simulink model "V1_Grid_Forming_corrected_dq_2022"  (R2022b)
settings: Solver=VariableStepAuto  StartTime=0.0  StopTime=2000e-3  RelTol=1e-3
InitFcn:
  | %% Initialize twist parameters
  | source_V = 0;
  | Ts = 1e-7;
  | 
  | % set the PID parameters
  | Kp = 0.000215;
  | Ti = 7.5175e-5;
  | Td = 0.0;
  | N  = 0.0;
  | Kd = 0.0;
  | 
  | 
  | %Low side parameters
  | twist_low_side_L = 33e-6;
  | twist_low_side_rL = 20e-3; %Modified
  | twist_low_side_C = 47e-6 + 3*4.7e-6;
  | twist_low_side_C_electrolytic = 47e-6;
  | twist_low_side_C_ceramic = 3*4.7e-6;
  | twist_low_side_rC = 700e-3;
  | twist_low_side_rC_ceramic = 0;
  | twist_low_side_adc_R = 150e3+470;
  | 
  | %High side parameters
  | twist_high_side_C = 33e-6*4 + 4.7e-6*12;
  | twist_high_side_rC = 0.1;
  | twist_high_side_adc_R = 1/(1/2e6 + 1/2e6 + 1/(330e3+5.6e3));
  | twist_high_side_feeder_R = 47e3+4.7e3;
  | R_parallel = 1/(1/twist_high_side_adc_R + 1/twist_high_side_feeder_R);
  | tau_VCC = 0.204;
  | tau_desactive = 0.2;
  | twist_R_VCC = (tau_VCC/twist_high_side_C  - twist_high_side_rC)/(1-(tau_VCC/twist_high_side_C - twist_high_side_rC)/R_parallel);
  | 
  | %High side feeder current
  | %load('feeder_current.mat');
  | feeder_VHigh_min = 12;
  | feeder_VHigh_spacing = 6;
  | feeder_duty_min = 0.1;
  | feeder_duty_spacing = 0.4;
  | feeder_Vth_stop = 8.9;
  | feeder_Vth_start = 9.7;
  | feeder_current_upper_rate_limit = 0.386/(20e-3);
  | feeder_current_lower_rate_limit = -500;
  | 
  | %MOSFET parameters
  | twist_FET_Ron = 0.016;
  | twist_FET_Lon = 0;
  | twist_FET_Rd = 0.006;
  | twist_FET_Vf = 0.7;
  | twist_FET_Rs = 1e10;
  | twist_FET_Cs = inf;
  | twist_FET_Clow_Ron = 220e-3;
  | twist_FET_Clow_Rd = 45e-3; %Modified
  | twist_FET_Clow_Vf = 0.7; %Modified
  | 
  | 
  | %Schottky diode parameters
  | twist_shottky_Ron = 0.48; %Modified
  | twist_shottky_Vf = 0.28; %Modified
  | twist_shottky_Rs = 1e10;
  | twist_shottky_Cs = inf;
  | 
  | %PWM generation
  | twist_freq_switching = 200e3; %carry switching frequency
  | twist_period_switching = 1/twist_freq_switching; %carry switching period
  | twist_pwm_resolution = 100e-9; %resolution of the PWM generator - increasing it reduces simulation time
  | twist_duty_cycle_min = 0; %minimum duty cycle
  | twist_duty_cycle_max = 1; %maximum duty cycle
  | twist_dead_time = 200e-9; %duty cycle positive dead time
  | 
  | % Initialize times and frequencies
  | twist_freq_data_sampling = 20e3; %data sampling frequency
  | twist_data_sampling_period = 1/twist_freq_data_sampling; %data sampling delay
  | twist_data_acquisition_delay = 50e-9; %data acquisition at the peak of the carry
undefined symbols (not defined in the file): DiscIntNeverNeededParam, gcbh, sps_rtmsupport, twist_low_side_lC
libraries: spsSeriesRLCBranchLib x13, spsTriangleGeneratorLib x6, spsMosfetLib x6, slpidlib x4, spsCurrentMeasurementLib x4, spsControlledCurrentSourceLib x3, spsVoltageMeasurementLib x3, eeTransforms x2, dspstat3 x2, spsIdealSwitchLib x2, spsDiodeLib x2, spspowerguiLib x2
(part 1 of 2)
settings Model: Creator=ABS_Lab  LastModifiedBy=ABS_Lab

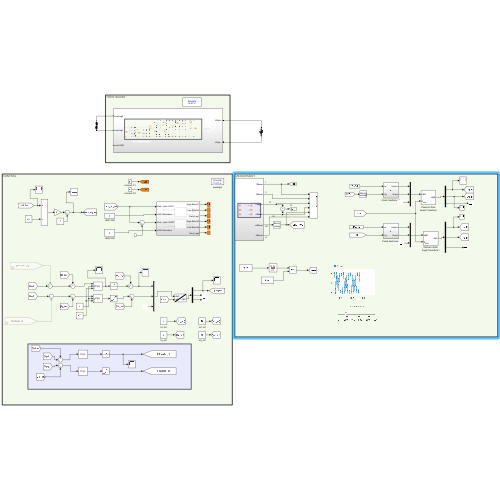
[thumbnail: Simulink's stored preview of the top-level diagram]
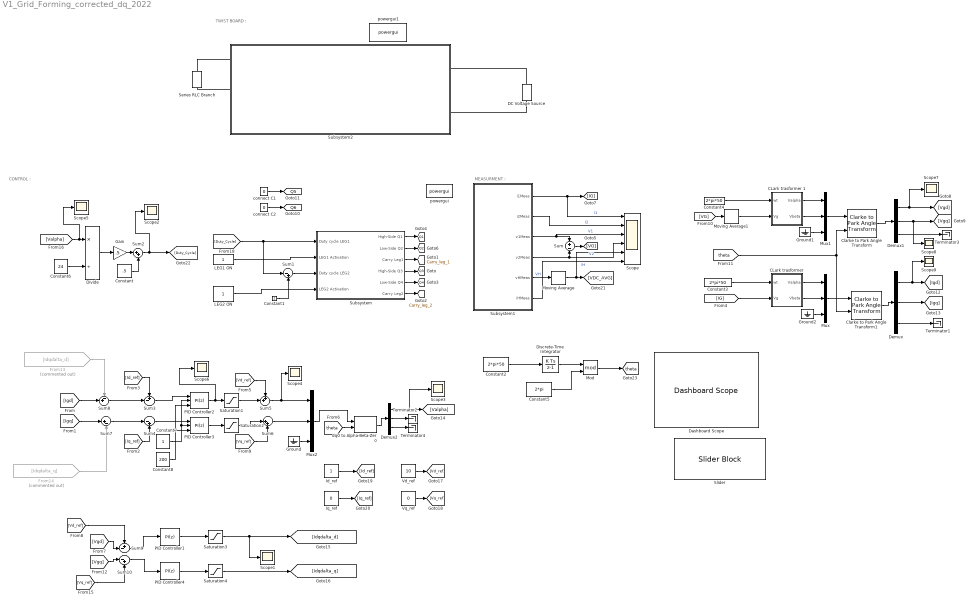
== system V1_Grid_Forming_corrected_dq_2022 ==
  note: TWIST BOARD :
  note: CONTROL :
  note: MEASURMENT :
  "CLark trasformer " : Subsystem
  CLark trasformer 1 : Subsystem
  Clarke to Park Angle Transform : eeTransforms/Clarke to Park Angle Transform  AxisAlignment=Q-axis
      settings: LibrarySourceBlock=|
      | ee_sl_lib/Mathematical
      | Transforms/Clarke to Park
      | Angle Transform
  Clarke to Park Angle Transform1 : eeTransforms/Clarke to Park Angle Transform  AxisAlignment=Q-axis
      settings: LibrarySourceBlock=|
      | ee_sl_lib/Mathematical
      | Transforms/Clarke to Park
      | Angle Transform
  Constant : Constant  Value=.5
  Constant1 : Constant
  Constant2 : Constant  Value=2*pi*50
  Constant3 : Constant  Value=2*pi*50
  Constant4 : Constant  Value=2*pi*50
  Constant5 : Constant  Value=2*pi
  Constant6 : Constant  Value=24
  Constant7 : Constant
  Constant8 : Constant  Value=200
  DC Voltage Source : spsDCVoltageSourceLib/DC Voltage Source  Amplitude=24  Measurements=None
  Dashboard Scope : DashboardScope  TimeSpan=0.080000000000000002  Ymin=-20  Ymax=20
  Demux : Demux  Outputs=3
  Demux1 : Demux  Outputs=3
  Demux2 : Demux  Outputs=3
  Discrete-Time Integrator : DiscreteIntegrator  SampleTime=-1  ICPrevOutput=DiscIntNeverNeededParam  ICPrevScaledInput=DiscIntNeverNeededParam
  Divide : Product  Inputs=*/
  From13 : From  Commented=on  GotoTag=Idqdalta_d
  From14 : From  Commented=on  GotoTag=Idqdalta_q
  Gain : Gain  Gain=.5
  Ground : Ground
  Ground1 : Ground
  Ground2 : Ground
  Id_ref : Constant
  Iq_ref : Constant  Value=0
  LEG1 ON : Constant
  LEG2 ON : Constant
  Mod : Math  Operator=mod
  Moving Average : dspstat3/Moving Average  Method=Sliding window  ForgettingFactorPort=off  SpecifyWindowLength=on  WindowLength=4  OverlapLength=3  AllowArbitraryInputLength=off  ForgettingFactor=0.9  SimulateUsing=Code generation
  Moving Average1 : dspstat3/Moving Average  Method=Sliding window  ForgettingFactorPort=off  SpecifyWindowLength=on  WindowLength=15  OverlapLength=14  AllowArbitraryInputLength=off  ForgettingFactor=0.9  SimulateUsing=Code generation
  Mux : Mux  Inputs=3
  Mux1 : Mux  Inputs=3
  Mux2 : Mux  Inputs=3
  PID Controller1 : slpidlib/PID Controller  Controller=PI  Form=Parallel  TimeDomain=Discrete-time  UseExternalTs=off  SampleTime=-1  IntegratorMethod=Forward Euler  FilterMethod=Forward Euler  ControllerParametersSource=internal  P=.01  I=3000  UseKiTs=off  D=0  N=100  UseFilter=on  TunerSelectOption=Transfer Function Based (PID Tuner App)  InitialConditionSource=internal  InitialConditionForIntegrator=0  InitialConditionForFilter=0  DifferentiatorICPrevScaledInput=0  ExternalReset=none  TrackingMode=off  Kt=1  LimitOutput=off  SatLimitsSource=internal  UpperSaturationLimit=inf  LowerSaturationLimit=-inf  LinearizeAsGain=on  AntiWindupMode=none  Kb=1  LimitIntegrator=off  UpperIntegratorSaturationLimit=inf  LowerIntegratorSaturationLimit=-inf  POutMin=[]  POutMax=[]  IOutMin=[]  IOutMax=[]  DOutMin=[]  DOutMax=[]  NOutMin=[]  NOutMax=[]  SumOutMin=[]  SumOutMax=[]  SaturationOutMin=[]  SaturationOutMax=[]  PParamMin=[]  PParamMax=[]  IParamMin=[]  IParamMax=[]  DParamMin=[]  DParamMax=[]  NParamMin=[]  NParamMax=[]  KbParamMin=[]  KbParamMax=[]  KtParamMin=[]  KtParamMax=[]  KbOutMin=[]  KbOutMax=[]  KtOutMin=[]  KtOutMax=[]  IntegratorOutMin=[]  IntegratorOutMax=[]  FilterOutMin=[]  FilterOutMax=[]  SumI1OutMin=[]  SumI1OutMax=[]  SumI2OutMin=[]  SumI2OutMax=[]  SumI3OutMin=[]  SumI3OutMax=[]  SumI4OutMin=[]  SumI4OutMax=[]  SumDOutMin=[]  SumDOutMax=[]  DifferentiatorOutMin=[]  DifferentiatorOutMax=[]  FilterDiffOutCoefMin=[]  FilterDiffOutCoefMax=[]  ReciprocalOutMin=[]  ReciprocalOutMax=[]  SumDenOutMin=[]  SumDenOutMax=[]  SumNumOutMin=[]  SumNumOutMax=[]  DivideOutMin=[]  DivideOutMax=[]  UdiffTsProdOutMin=[]  UdiffTsProdOutMax=[]  NTsProdOutMin=[]  NTsProdOutMax=[]  UintegralTsProdOutMin=[]  UintegralTsProdOutMax=[]  UngainTsProdOutMin=[]  UngainTsProdOutMax=[]  ClampingZeroOutDataTypeStr=Inherit: Inherit via back propagation  ClampingZeroOutMin=[]  ClampingZeroOutMax=[]  FilterDenConstantOutDataTypeStr=Inherit: Inherit via back propagation  FilterDenConstantOutMin=[]  FilterDenConstantOutMax=[]  PCopyOutDataTypeStr=Inherit: Inherit via back propagation  PCopyOutMin=[]  PCopyOutMax=[]  NCopyOutDataTypeStr=Inherit: Inherit via back propagation  NCopyOutMin=[]  NCopyOutMax=[]  IntegratorContinuousStateAttributes=''  IntegratorStateMustResolveToSignalObject=off  IntegratorRTWStateStorageClass=Auto  FilterContinuousStateAttributes=''  FilterStateMustResolveToSignalObject=off  FilterRTWStateStorageClass=Auto  ParallelPVariant=InternalParameters  IdealPVariant=Disabled  IVariant=InternalParameters  DVariant=Disabled  IntegratorVariant=Discrete  SatVariant=Disabled  AWVariant=Passthrough  PCopyVariant=Disabled  TRVariant=Disabled  FdbkBlocksVariant=Forward  IdealPFdbkVariant=Disabled  SatFdbkVariant=Disabled  DerivativeFilterVariant=Disabled  NVariant=Disabled  NCopyVariant=Disabled_SignalSpec  FilterICVariant=Disabled  IntegratorICVariant=InternalICs  ExternalResetVariant=Disabled  TRSumVariant=Passthrough  SumFdbkVariant=Disabled  SumVariant=Sum_PI  TsampFilterVariant=InternalTs  TsampNgainVariant=Passthrough  TsampIntegralVariant=Passthrough  ExternalSaturationOutDataTypeStr=Inherit: Same as second input
  PID Controller2 : slpidlib/PID Controller  Controller=PI  Form=Parallel  TimeDomain=Discrete-time  UseExternalTs=off  SampleTime=Ts*1000  IntegratorMethod=Forward Euler  FilterMethod=Forward Euler  ControllerParametersSource=external  P=.1  I=2000  UseKiTs=off  D=0  N=100  UseFilter=on  TunerSelectOption=Transfer Function Based (PID Tuner App)  InitialConditionSource=internal  InitialConditionForIntegrator=0  InitialConditionForFilter=0  DifferentiatorICPrevScaledInput=0  ExternalReset=none  TrackingMode=off  Kt=1  LimitOutput=off  SatLimitsSource=internal  UpperSaturationLimit=inf  LowerSaturationLimit=-inf  LinearizeAsGain=on  AntiWindupMode=none  Kb=1  LimitIntegrator=off  UpperIntegratorSaturationLimit=inf  LowerIntegratorSaturationLimit=-inf  POutMin=[]  POutMax=[]  IOutMin=[]  IOutMax=[]  DOutMin=[]  DOutMax=[]  NOutMin=[]  NOutMax=[]  SumOutMin=[]  SumOutMax=[]  SaturationOutMin=[]  SaturationOutMax=[]  PParamMin=[]  PParamMax=[]  IParamMin=[]  IParamMax=[]  DParamMin=[]  DParamMax=[]  NParamMin=[]  NParamMax=[]  KbParamMin=[]  KbParamMax=[]  KtParamMin=[]  KtParamMax=[]  KbOutMin=[]  KbOutMax=[]  KtOutMin=[]  KtOutMax=[]  IntegratorOutMin=[]  IntegratorOutMax=[]  FilterOutMin=[]  FilterOutMax=[]  SumI1OutMin=[]  SumI1OutMax=[]  SumI2OutMin=[]  SumI2OutMax=[]  SumI3OutMin=[]  SumI3OutMax=[]  SumI4OutMin=[]  SumI4OutMax=[]  SumDOutMin=[]  SumDOutMax=[]  DifferentiatorOutMin=[]  DifferentiatorOutMax=[]  FilterDiffOutCoefMin=[]  FilterDiffOutCoefMax=[]  ReciprocalOutMin=[]  ReciprocalOutMax=[]  SumDenOutMin=[]  SumDenOutMax=[]  SumNumOutMin=[]  SumNumOutMax=[]  DivideOutMin=[]  DivideOutMax=[]  UdiffTsProdOutMin=[]  UdiffTsProdOutMax=[]  NTsProdOutMin=[]  NTsProdOutMax=[]  UintegralTsProdOutMin=[]  UintegralTsProdOutMax=[]  UngainTsProdOutMin=[]  UngainTsProdOutMax=[]  ClampingZeroOutDataTypeStr=Inherit: Inherit via back propagation  ClampingZeroOutMin=[]  ClampingZeroOutMax=[]  FilterDenConstantOutDataTypeStr=Inherit: Inherit via back propagation  FilterDenConstantOutMin=[]  FilterDenConstantOutMax=[]  PCopyOutDataTypeStr=Inherit: Inherit via back propagation  PCopyOutMin=[]  PCopyOutMax=[]  NCopyOutDataTypeStr=Inherit: Inherit via back propagation  NCopyOutMin=[]  NCopyOutMax=[]  IntegratorContinuousStateAttributes=''  IntegratorStateMustResolveToSignalObject=off  IntegratorRTWStateStorageClass=Auto  FilterContinuousStateAttributes=''  FilterStateMustResolveToSignalObject=off  FilterRTWStateStorageClass=Auto  ParallelPVariant=ExternalParameters  IdealPVariant=Disabled  IVariant=ExternalParameters  DVariant=Disabled  IntegratorVariant=Discrete  SatVariant=Disabled  AWVariant=Passthrough  PCopyVariant=Disabled  TRVariant=Disabled  FdbkBlocksVariant=Forward  IdealPFdbkVariant=Disabled  SatFdbkVariant=Disabled  DerivativeFilterVariant=Disabled  NVariant=Disabled  NCopyVariant=Disabled_SignalSpec  FilterICVariant=Disabled  IntegratorICVariant=InternalICs  ExternalResetVariant=Disabled  TRSumVariant=Passthrough  SumFdbkVariant=Disabled  SumVariant=Sum_PI  TsampFilterVariant=InternalTs  TsampNgainVariant=Passthrough  TsampIntegralVariant=Passthrough  ExternalSaturationOutDataTypeStr=Inherit: Same as second input
  PID Controller3 : slpidlib/PID Controller  Controller=PI  Form=Parallel  TimeDomain=Discrete-time  UseExternalTs=off  SampleTime=Ts*1000  IntegratorMethod=Forward Euler  FilterMethod=Forward Euler  ControllerParametersSource=external  P=.1  I=100  UseKiTs=off  D=0  N=100  UseFilter=on  TunerSelectOption=Transfer Function Based (PID Tuner App)  InitialConditionSource=internal  InitialConditionForIntegrator=0  InitialConditionForFilter=0  DifferentiatorICPrevScaledInput=0  ExternalReset=none  TrackingMode=off  Kt=1  LimitOutput=off  SatLimitsSource=internal  UpperSaturationLimit=inf  LowerSaturationLimit=-inf  LinearizeAsGain=on  AntiWindupMode=none  Kb=1  LimitIntegrator=off  UpperIntegratorSaturationLimit=inf  LowerIntegratorSaturationLimit=-inf  POutMin=[]  POutMax=[]  IOutMin=[]  IOutMax=[]  DOutMin=[]  DOutMax=[]  NOutMin=[]  NOutMax=[]  SumOutMin=[]  SumOutMax=[]  SaturationOutMin=[]  SaturationOutMax=[]  PParamMin=[]  PParamMax=[]  IParamMin=[]  IParamMax=[]  DParamMin=[]  DParamMax=[]  NParamMin=[]  NParamMax=[]  KbParamMin=[]  KbParamMax=[]  KtParamMin=[]  KtParamMax=[]  KbOutMin=[]  KbOutMax=[]  KtOutMin=[]  KtOutMax=[]  IntegratorOutMin=[]  IntegratorOutMax=[]  FilterOutMin=[]  FilterOutMax=[]  SumI1OutMin=[]  SumI1OutMax=[]  SumI2OutMin=[]  SumI2OutMax=[]  SumI3OutMin=[]  SumI3OutMax=[]  SumI4OutMin=[]  SumI4OutMax=[]  SumDOutMin=[]  SumDOutMax=[]  DifferentiatorOutMin=[]  DifferentiatorOutMax=[]  FilterDiffOutCoefMin=[]  FilterDiffOutCoefMax=[]  ReciprocalOutMin=[]  ReciprocalOutMax=[]  SumDenOutMin=[]  SumDenOutMax=[]  SumNumOutMin=[]  SumNumOutMax=[]  DivideOutMin=[]  DivideOutMax=[]  UdiffTsProdOutMin=[]  UdiffTsProdOutMax=[]  NTsProdOutMin=[]  NTsProdOutMax=[]  UintegralTsProdOutMin=[]  UintegralTsProdOutMax=[]  UngainTsProdOutMin=[]  UngainTsProdOutMax=[]  ClampingZeroOutDataTypeStr=Inherit: Inherit via back propagation  ClampingZeroOutMin=[]  ClampingZeroOutMax=[]  FilterDenConstantOutDataTypeStr=Inherit: Inherit via back propagation  FilterDenConstantOutMin=[]  FilterDenConstantOutMax=[]  PCopyOutDataTypeStr=Inherit: Inherit via back propagation  PCopyOutMin=[]  PCopyOutMax=[]  NCopyOutDataTypeStr=Inherit: Inherit via back propagation  NCopyOutMin=[]  NCopyOutMax=[]  IntegratorContinuousStateAttributes=''  IntegratorStateMustResolveToSignalObject=off  IntegratorRTWStateStorageClass=Auto  FilterContinuousStateAttributes=''  FilterStateMustResolveToSignalObject=off  FilterRTWStateStorageClass=Auto  ParallelPVariant=ExternalParameters  IdealPVariant=Disabled  IVariant=ExternalParameters  DVariant=Disabled  IntegratorVariant=Discrete  SatVariant=Disabled  AWVariant=Passthrough  PCopyVariant=Disabled  TRVariant=Disabled  FdbkBlocksVariant=Forward  IdealPFdbkVariant=Disabled  SatFdbkVariant=Disabled  DerivativeFilterVariant=Disabled  NVariant=Disabled  NCopyVariant=Disabled_SignalSpec  FilterICVariant=Disabled  IntegratorICVariant=InternalICs  ExternalResetVariant=Disabled  TRSumVariant=Passthrough  SumFdbkVariant=Disabled  SumVariant=Sum_PI  TsampFilterVariant=InternalTs  TsampNgainVariant=Passthrough  TsampIntegralVariant=Passthrough  ExternalSaturationOutDataTypeStr=Inherit: Same as second input
  PID Controller4 : slpidlib/PID Controller  Controller=PI  Form=Parallel  TimeDomain=Discrete-time  UseExternalTs=off  SampleTime=-1  IntegratorMethod=Forward Euler  FilterMethod=Forward Euler  ControllerParametersSource=internal  P=.01  I=3000  UseKiTs=off  D=0  N=100  UseFilter=on  TunerSelectOption=Transfer Function Based (PID Tuner App)  InitialConditionSource=internal  InitialConditionForIntegrator=0  InitialConditionForFilter=0  DifferentiatorICPrevScaledInput=0  ExternalReset=none  TrackingMode=off  Kt=1  LimitOutput=off  SatLimitsSource=internal  UpperSaturationLimit=inf  LowerSaturationLimit=-inf  LinearizeAsGain=on  AntiWindupMode=none  Kb=1  LimitIntegrator=off  UpperIntegratorSaturationLimit=inf  LowerIntegratorSaturationLimit=-inf  POutMin=[]  POutMax=[]  IOutMin=[]  IOutMax=[]  DOutMin=[]  DOutMax=[]  NOutMin=[]  NOutMax=[]  SumOutMin=[]  SumOutMax=[]  SaturationOutMin=[]  SaturationOutMax=[]  PParamMin=[]  PParamMax=[]  IParamMin=[]  IParamMax=[]  DParamMin=[]  DParamMax=[]  NParamMin=[]  NParamMax=[]  KbParamMin=[]  KbParamMax=[]  KtParamMin=[]  KtParamMax=[]  KbOutMin=[]  KbOutMax=[]  KtOutMin=[]  KtOutMax=[]  IntegratorOutMin=[]  IntegratorOutMax=[]  FilterOutMin=[]  FilterOutMax=[]  SumI1OutMin=[]  SumI1OutMax=[]  SumI2OutMin=[]  SumI2OutMax=[]  SumI3OutMin=[]  SumI3OutMax=[]  SumI4OutMin=[]  SumI4OutMax=[]  SumDOutMin=[]  SumDOutMax=[]  DifferentiatorOutMin=[]  DifferentiatorOutMax=[]  FilterDiffOutCoefMin=[]  FilterDiffOutCoefMax=[]  ReciprocalOutMin=[]  ReciprocalOutMax=[]  SumDenOutMin=[]  SumDenOutMax=[]  SumNumOutMin=[]  SumNumOutMax=[]  DivideOutMin=[]  DivideOutMax=[]  UdiffTsProdOutMin=[]  UdiffTsProdOutMax=[]  NTsProdOutMin=[]  NTsProdOutMax=[]  UintegralTsProdOutMin=[]  UintegralTsProdOutMax=[]  UngainTsProdOutMin=[]  UngainTsProdOutMax=[]  ClampingZeroOutDataTypeStr=Inherit: Inherit via back propagation  ClampingZeroOutMin=[]  ClampingZeroOutMax=[]  FilterDenConstantOutDataTypeStr=Inherit: Inherit via back propagation  FilterDenConstantOutMin=[]  FilterDenConstantOutMax=[]  PCopyOutDataTypeStr=Inherit: Inherit via back propagation  PCopyOutMin=[]  PCopyOutMax=[]  NCopyOutDataTypeStr=Inherit: Inherit via back propagation  NCopyOutMin=[]  NCopyOutMax=[]  IntegratorContinuousStateAttributes=''  IntegratorStateMustResolveToSignalObject=off  IntegratorRTWStateStorageClass=Auto  FilterContinuousStateAttributes=''  FilterStateMustResolveToSignalObject=off  FilterRTWStateStorageClass=Auto  ParallelPVariant=InternalParameters  IdealPVariant=Disabled  IVariant=InternalParameters  DVariant=Disabled  IntegratorVariant=Discrete  SatVariant=Disabled  AWVariant=Passthrough  PCopyVariant=Disabled  TRVariant=Disabled  FdbkBlocksVariant=Forward  IdealPFdbkVariant=Disabled  SatFdbkVariant=Disabled  DerivativeFilterVariant=Disabled  NVariant=Disabled  NCopyVariant=Disabled_SignalSpec  FilterICVariant=Disabled  IntegratorICVariant=InternalICs  ExternalResetVariant=Disabled  TRSumVariant=Passthrough  SumFdbkVariant=Disabled  SumVariant=Sum_PI  TsampFilterVariant=InternalTs  TsampNgainVariant=Passthrough  TsampIntegralVariant=Passthrough  ExternalSaturationOutDataTypeStr=Inherit: Same as second input
  Saturation1 : Saturate  UpperLimit=24  LowerLimit=-24
  Saturation2 : Saturate  UpperLimit=24  LowerLimit=-24
  Saturation3 : Saturate  UpperLimit=10  LowerLimit=-10
  Saturation4 : Saturate  UpperLimit=10  LowerLimit=-10
  Scope : Scope  NumInputPorts=6
  Scope{1..9} (9 alike) : Scope
  Series RLC Branch : spsSeriesRLCBranchLib/Series RLC Branch  LConnTagsString=__new0  RConnTagsString=__new0  BranchType=RL  Resistance=10  Inductance=100e-8  SetiL0=off  InitialCurrent=0  Capacitance=1e-6  Setx0=off  InitialVoltage=0  Measurements=None
  Slider : SliderBlock  ScaleMax=1000
  Subsystem : Subsystem
  Subsystem1 : Subsystem
  Subsystem2 : Subsystem
  Sum : Sum  Inputs=+|-
  Sum1 : Sum  Inputs=|-+
  Sum10 : Sum  Inputs=|-+
  Sum2 : Sum  Inputs=|++
  Sum3 : Sum  Inputs=+-|
  Sum4 : Sum  Inputs=|-+
  Sum5 : Sum  Inputs=++|
  Sum6 : Sum  Inputs=|++
  Sum7 : Sum  Inputs=|+-
  Sum8 : Sum  Inputs=-+|
  Sum9 : Sum  Inputs=+-|
  Terminator{1..4} (4 alike) : Terminator
  Vd_ref : Constant  Value=10
  Vq_ref : Constant  Value=0
  connect C1 : Constant  Value=0
  connect C2 : Constant  Value=0
  dq0 to Alpha-Beta-Zero : spsdq0toAlphaBetaZeroLib/dq0 to Alpha-Beta-Zero  Alignment=90 degrees behind phase A axis
  powergui : spspowerguiLib/powergui  Priority=1  SimulationMode=Discrete  SampleTime=Ts  frequency=60  Iterations=50  frequencyindice=0  Pbase=100e6  ErrMax=1e-4  UnitsV=kV  UnitsW=MW  buscounter=0  FunctionMessages=off  echomessages=off  EnableUseOfTLC=off  CurrentSourceSwitches=off  DisableSnubberDevices=off  DisableRonSwitches=off  DisableVfSwitches=off  DisplayEquations=off  AutomaticDiscreteSolvers=off  SolverType=Tustin/Backward Euler (TBE)  Interpol=off  ExternalGateDelay=off  methode=off  Ts=100  x0status=blocks  SPID=on  SwTol=0  HookPort=off  NonlinearTolerance=1e-4  nMaxIteration=100  ContinueOnMaxIteration=off  RestoreLinks=warning  ResistiveCurrentMeasurement=off  Frange=[0:2:500]  Ylog=off  Xlog=on  ShowGrid=off  save=off  variable=ZData  structure=0  ZoomFFT=off  StartTime=0.0  cycles=1  DisplayStyle=1  fundamental=60  FreqAxis=off  MaxFrequency=1000  frequencyindicesteady=1  RmsSteady=1  display=off
  powergui1 : spspowerguiLib/powergui  Priority=1  SimulationMode=Discrete  SampleTime=Ts  frequency=60  Iterations=50  frequencyindice=60  Pbase=100e6  ErrMax=1e-4  UnitsV=kV  UnitsW=MW  buscounter=0  FunctionMessages=off  echomessages=off  EnableUseOfTLC=off  CurrentSourceSwitches=off  DisableSnubberDevices=off  DisableRonSwitches=off  DisableVfSwitches=off  DisplayEquations=off  AutomaticDiscreteSolvers=off  SolverType=Tustin/Backward Euler (TBE)  Interpol=off  ExternalGateDelay=off  methode=off  Ts=100  x0status=blocks  SPID=on  SwTol=0  HookPort=off  NonlinearTolerance=1e-4  nMaxIteration=100  ContinueOnMaxIteration=off  RestoreLinks=warning  ResistiveCurrentMeasurement=off  Frange=[0:2:500]  Ylog=off  Xlog=on  ShowGrid=off  save=off  variable=ZData  structure=0  ZoomFFT=off  StartTime=0.0  cycles=1  DisplayStyle=1  fundamental=60  FreqAxis=off  MaxFrequency=1000  frequencyindicesteady=1  RmsSteady=1  display=off
  tag scope: Carry_leg_1=global, Carry_leg_2=global, Q1=global, Q2=global, Q3=global, Q4=global, Q5=global, Q6=global, theta=global
  wires:
  Sum1/1 -> Subsystem/3(Duty cycle LEG2)
  connect C1/1 -> [Q5]
  LEG1 ON/1 -> Subsystem/2(LEG1 Activation)
  Subsystem/3(Carry Leg1) -> [Carry_leg_1]
  Subsystem1/3(v1Meas) -> Scope/3, Sum/1  "V1"
  LEG2 ON/1 -> Subsystem/4("LEG2 Activation ")
  [Duty_Cycle] -> Sum1/1, Subsystem/1(Duty cycle LEG1)
  connect C2/1 -> [Q6]
  Subsystem/2(Low-Side Q2) -> [Q2]
  Subsystem/5(Low-Side Q4) -> [Q4]
  Subsystem1/6(iHMeas) -> Scope/6  "IH"
  Subsystem/1(High-Side Q1) -> [Q1]
  Subsystem/6(Carry Leg2) -> [Carry_leg_2]
  Constant1/1 -> Sum1/2
  Subsystem1/2(i2Meas) -> Scope/2  "I2"
  Subsystem/4(High-Side Q3) -> [Q3]
  Subsystem1/4(v2Meas) -> Scope/4, Sum/2  "V2"
  Demux1/1 -> Scope7/1, [Vgd]
  CLark trasformer 1/2(Vbeta) -> Mux1/2
  [VG] -> Moving Average1/1
  CLark trasformer 1/1(Valpha) -> Mux1/1
  Constant4/1 -> CLark trasformer 1/1(wt)
  Clarke to Park Angle Transform/1 -> Demux1/1
  Mux1/1 -> Clarke to Park Angle Transform/1
  Demux1/2 -> Scope8/1, [Vgq]
  [theta] -> Clarke to Park Angle Transform1/2, Clarke to Park Angle Transform/2
  Demux1/3 -> Terminator3/1
  Sum/1 -> [VG]
  Demux/2 -> [Igq]
  "CLark trasformer "/1(Valpha) -> Mux/1
  Demux/1 -> Scope9/1, [Igd]
  "CLark trasformer "/2(Vbeta) -> Mux/2
  Constant3/1 -> "CLark trasformer "/1(wt)
  Demux/3 -> Terminator1/1
  Clarke to Park Angle Transform1/1 -> Demux/1
  [IG] -> "CLark trasformer "/2(Vg)
  Mux/1 -> Clarke to Park Angle Transform1/1
  Subsystem1/1(i1Meas) -> Scope/1, [IG]  "I1"
  Sum7/1 -> Sum4/1
  Sum5/1 -> Scope4/1, Mux2/1
  Saturation2/1 -> Sum6/1
  From14/1 -> Sum7/2
  Demux2/2 -> Terminator2/1
  Sum6/1 -> Mux2/2
  Saturation1/1 -> Sum5/2
  PID Controller3/1 -> Saturation2/1
  Demux2/1 -> Scope3/1, [Valpha]
  Sum4/1 -> PID Controller3/1
  Mux2/1 -> dq0 to Alpha-Beta-Zero/1
  Sum3/1 -> PID Controller2/1
  dq0 to Alpha-Beta-Zero/1 -> Demux2/1
  From13/1 -> Sum8/1
  Sum8/1 -> Sum3/2
  [theta] -> dq0 to Alpha-Beta-Zero/2
  Demux2/3 -> Terminator4/1
  PID Controller2/1 -> Scope6/1, Saturation1/1
  [Igd] -> Sum8/2
  [Igq] -> Sum7/1
  [Vd_ref] -> Sum9/1
  PID Controller1/1 -> Saturation3/1
  Saturation3/1 -> Scope1/1, [Idqdalta_d]
  PID Controller4/1 -> Saturation4/1
  Saturation4/1 -> [Idqdalta_q]
  Sum9/1 -> PID Controller1/1
  [Vgd] -> Sum9/2
  [Vgq] -> Sum10/1
  Sum10/1 -> PID Controller4/1
  [Vq_ref] -> Sum10/2
  Vd_ref/1 -> [Vd_ref]
  Vq_ref/1 -> [Vq_ref]
  Id_ref/1 -> [Id_ref]
  Iq_ref/1 -> [Iq_ref]
  [Id_ref] -> Sum3/1
  [Iq_ref] -> Sum4/2
  [Vd_ref] -> Sum5/1
  Ground/1 -> Mux2/3
  [Vq_ref] -> Sum6/2
  [Valpha] -> Scope5/1, Divide/1
  Subsystem1/5(vHMeas) -> Moving Average/1  "VH"
  Moving Average/1 -> Scope/5, [VDC_AVG]
  Constant6/1 -> Divide/2
  Divide/1 -> Gain/1
  Gain/1 -> Sum2/1
  Constant/1 -> Sum2/2
  Sum2/1 -> Scope2/1, [Duty_Cycle]
  Ground1/1 -> Mux1/3
  Ground2/1 -> Mux/3
  Mod/1 -> [theta]
  Discrete-Time Integrator/1 -> Mod/1
  Constant2/1 -> Discrete-Time Integrator/1
  Constant5/1 -> Mod/2
  Moving Average1/1 -> CLark trasformer 1/2(Vg)
  Constant7/1 -> PID Controller3/2, PID Controller2/2
  Constant8/1 -> PID Controller3/3, PID Controller2/3
  connections:
  DC Voltage Source/RConn1 -- Subsystem2/RConn1
  Series RLC Branch/LConn1 -- Subsystem2/LConn1
  Subsystem2/LConn2 -- Series RLC Branch/RConn1
  DC Voltage Source/LConn1 -- Subsystem2/RConn2

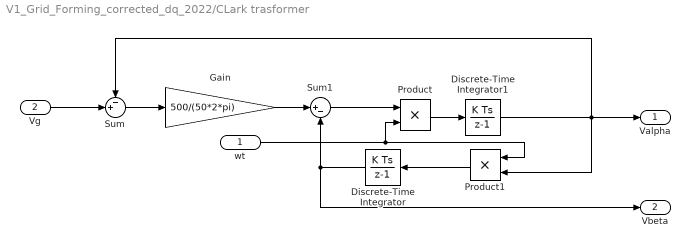
== system V1_Grid_Forming_corrected_dq_2022/CLark trasformer  ==
  wt : Inport
  Vg : Inport  Port=2
  Discrete-Time Integrator : DiscreteIntegrator  SampleTime=Ts*1000  ICPrevOutput=DiscIntNeverNeededParam  ICPrevScaledInput=DiscIntNeverNeededParam
  Discrete-Time Integrator1 : DiscreteIntegrator  SampleTime=Ts*1000  ICPrevOutput=DiscIntNeverNeededParam  ICPrevScaledInput=DiscIntNeverNeededParam
  Gain : Gain  Gain=500/(50*2*pi)
  Product : Product
  Product1 : Product
  Sum : Sum  Inputs=-+|
  Sum1 : Sum  Inputs=|+-
  Valpha : Outport
  Vbeta : Outport  Port=2
  wires:
  Product/1 -> Discrete-Time Integrator1/1
  Discrete-Time Integrator1/1 -> Valpha/1, Product1/2, Sum/1
  Discrete-Time Integrator/1 -> Vbeta/1, Sum1/2
  Gain/1 -> Sum1/1
  wt/1 -> Product1/1, Product/2
  Sum/1 -> Gain/1
  Sum1/1 -> Product/1
  Product1/1 -> Discrete-Time Integrator/1
  Vg/1 -> Sum/2

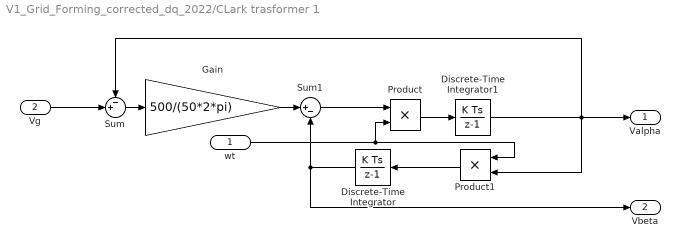
== system V1_Grid_Forming_corrected_dq_2022/CLark trasformer 1 ==
  wt : Inport
  Vg : Inport  Port=2
  Discrete-Time Integrator : DiscreteIntegrator  SampleTime=Ts*1e3  ICPrevOutput=DiscIntNeverNeededParam  ICPrevScaledInput=DiscIntNeverNeededParam
  Discrete-Time Integrator1 : DiscreteIntegrator  SampleTime=Ts*1e3  ICPrevOutput=DiscIntNeverNeededParam  ICPrevScaledInput=DiscIntNeverNeededParam
  Gain : Gain  Gain=500/(50*2*pi)
  Product : Product
  Product1 : Product
  Sum : Sum  Inputs=-+|
  Sum1 : Sum  Inputs=|+-
  Valpha : Outport
  Vbeta : Outport  Port=2
  wires:
  Vg/1 -> Sum/2
  Product1/1 -> Discrete-Time Integrator/1
  Sum1/1 -> Product/1
  Sum/1 -> Gain/1
  wt/1 -> Product/2, Product1/1
  Gain/1 -> Sum1/1
  Discrete-Time Integrator/1 -> Sum1/2, Vbeta/1
  Discrete-Time Integrator1/1 -> Sum/1, Product1/2, Valpha/1
  Product/1 -> Discrete-Time Integrator1/1

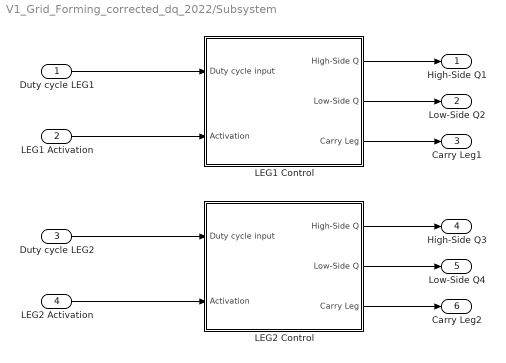
== system V1_Grid_Forming_corrected_dq_2022/Subsystem ==
  Duty cycle LEG1 : Inport
  LEG1 Activation : Inport  Port=2
  Duty cycle LEG2 : Inport  Port=3
  "LEG2 Activation " : Inport  Port=4
  "LEG1 Control " : Subsystem
  LEG2 Control : Subsystem
  High-Side Q1 : Outport
  Low-Side Q2 : Outport  Port=2
  Carry Leg1 : Outport  Port=3
  High-Side Q3 : Outport  Port=4
  Low-Side Q4 : Outport  Port=5
  Carry Leg2 : Outport  Port=6
  wires:
  "LEG1 Control "/3(Carry Leg) -> Carry Leg1/1
  LEG2 Control/1(High-Side Q) -> High-Side Q3/1
  Duty cycle LEG1/1 -> "LEG1 Control "/1(Duty cycle input)
  Duty cycle LEG2/1 -> LEG2 Control/1(Duty cycle input)
  LEG1 Activation/1 -> "LEG1 Control "/2(Activation)
  LEG2 Control/2(Low-Side Q) -> Low-Side Q4/1
  "LEG2 Activation "/1 -> LEG2 Control/2(Activation)
  LEG2 Control/3(Carry Leg) -> Carry Leg2/1
  "LEG1 Control "/1(High-Side Q) -> High-Side Q1/1
  "LEG1 Control "/2(Low-Side Q) -> Low-Side Q2/1

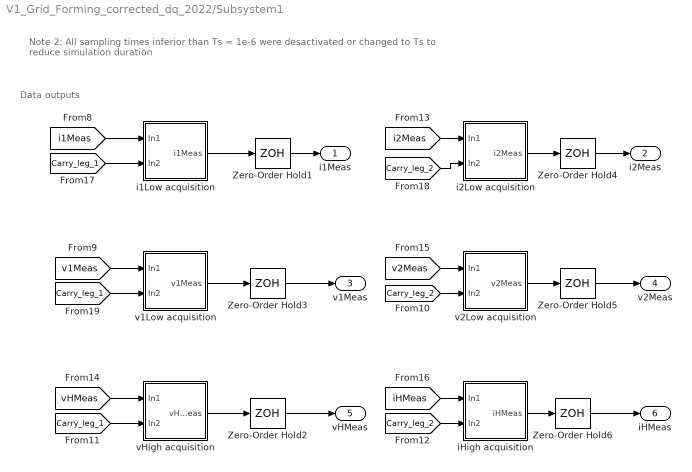
== system V1_Grid_Forming_corrected_dq_2022/Subsystem1 ==
  note: Note 2:
      | All sampling times inferior than Ts = 1e-6 were desactivated or changed to Ts to reduce simulation duration
  note: Data outputs
  Zero-Order Hold{1..6} (6 alike) : ZeroOrderHold  SampleTime=twist_data_sampling_period
  i1Low acquisition : Subsystem
  i2Low acquisition : Subsystem
  iHigh acquisition : Subsystem
  v1Low acquisition : Subsystem
  v2Low acquisition : Subsystem
  vHigh acquisition : Subsystem
  i1Meas : Outport
  i2Meas : Outport  Port=2
  v1Meas : Outport  Port=3
  v2Meas : Outport  Port=4
  vHMeas : Outport  Port=5
  iHMeas : Outport  Port=6
  wires:
  [v2Meas] -> v2Low acquisition/1(In1)
  Zero-Order Hold4/1 -> i2Meas/1
  vHigh acquisition/1(vHMeas) -> Zero-Order Hold2/1
  [i1Meas] -> i1Low acquisition/1(In1)
  [Carry_leg_1] -> vHigh acquisition/2(In2)
  [Carry_leg_1] -> v1Low acquisition/2(In2)
  [vHMeas] -> vHigh acquisition/1(In1)
  [Carry_leg_1] -> i1Low acquisition/2(In2)
  [Carry_leg_2] -> v2Low acquisition/2(In2)
  [v1Meas] -> v1Low acquisition/1(In1)
  Zero-Order Hold5/1 -> v2Meas/1
  [iHMeas] -> iHigh acquisition/1(In1)
  [i2Meas] -> i2Low acquisition/1(In1)
  Zero-Order Hold1/1 -> i1Meas/1
  i2Low acquisition/1(i2Meas) -> Zero-Order Hold4/1
  Zero-Order Hold6/1 -> iHMeas/1
  i1Low acquisition/1(i1Meas) -> Zero-Order Hold1/1
  Zero-Order Hold2/1 -> vHMeas/1
  v1Low acquisition/1(v1Meas) -> Zero-Order Hold3/1
  [Carry_leg_2] -> iHigh acquisition/2(In2)
  [Carry_leg_2] -> i2Low acquisition/2(In2)
  Zero-Order Hold3/1 -> v1Meas/1
  iHigh acquisition/1(iHMeas) -> Zero-Order Hold6/1
  v2Low acquisition/1(v2Meas) -> Zero-Order Hold5/1

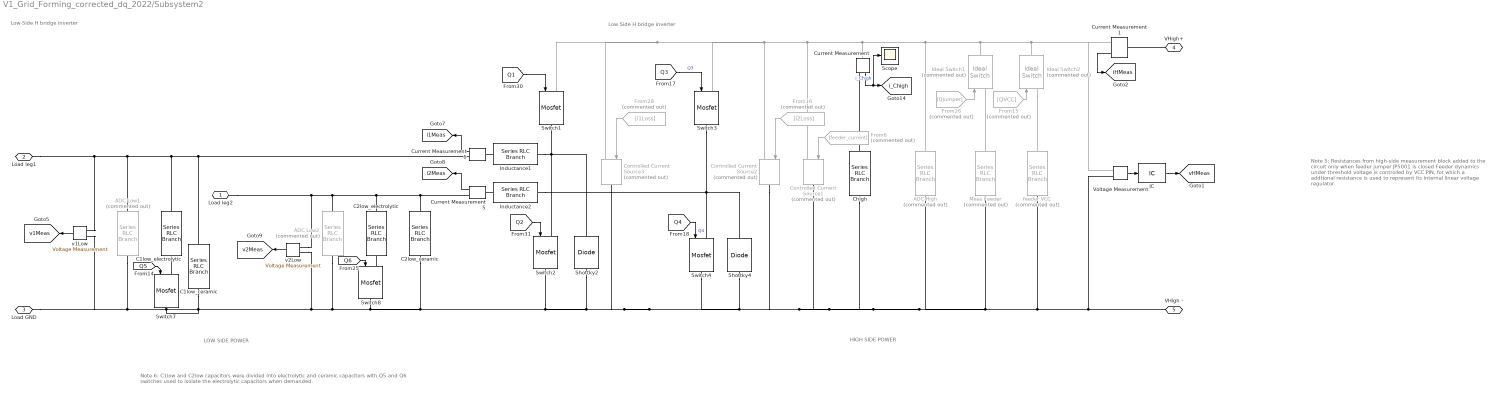
== system V1_Grid_Forming_corrected_dq_2022/Subsystem2 ==
  note: Note 5:
      |
      | Resistances from high-side measurement block added to the circuit only when feeder jumper JP5001 is closed
      |
      | Feeder dynamics under threshold voltage is controlled by VCC PIN, for which a addtional resistance is used to represent its internal linear voltage regulator
  note: Note 6:
      | C1low and C2low capacitors were divided into electrolytic and ceramic capacitors with Q5 and Q6 switches used to isolate the electrolytic capacitors when demanded.
  note: Low Side H bridge inverter
  note: LOW SIDE POWER
  note: HIGH SIDE POWER
  note: Low-Side H bridge inverter
  ADC High : spsSeriesRLCBranchLib/Series RLC Branch  Commented=on  LConnTagsString=__new0  RConnTagsString=__new0  BranchType=R  Resistance=twist_high_side_adc_R  Inductance=twist_low_side_L  SetiL0=off  InitialCurrent=0  Capacitance=1e-6  Setx0=off  InitialVoltage=0  Measurements=None
  ADC Low1 : spsSeriesRLCBranchLib/Series RLC Branch  Commented=on  LConnTagsString=__new0  RConnTagsString=__new0  BranchType=R  Resistance=twist_low_side_adc_R  Inductance=twist_low_side_L  SetiL0=off  InitialCurrent=0  Capacitance=1e-6  Setx0=off  InitialVoltage=0  Measurements=Branch voltage
  ADC Low2 : spsSeriesRLCBranchLib/Series RLC Branch  Commented=on  LConnTagsString=__new0  RConnTagsString=__new0  BranchType=R  Resistance=twist_low_side_adc_R  Inductance=twist_low_side_L  SetiL0=off  InitialCurrent=0  Capacitance=1e-6  Setx0=off  InitialVoltage=0  Measurements=Branch voltage
  C1low_ceramic : spsSeriesRLCBranchLib/Series RLC Branch  LConnTagsString=__new0  RConnTagsString=__new0  BranchType=C  Resistance=twist_low_side_rC  Inductance=1e-3  SetiL0=off  InitialCurrent=0  Capacitance=twist_low_side_C_ceramic  Setx0=off  InitialVoltage=source_V  Measurements=None
  C1low_electrolytic : spsSeriesRLCBranchLib/Series RLC Branch  LConnTagsString=__new0  RConnTagsString=__new0  BranchType=RC  Resistance=twist_low_side_rC  Inductance=twist_low_side_lC  SetiL0=off  InitialCurrent=0  Capacitance=twist_low_side_C_electrolytic  Setx0=off  InitialVoltage=source_V  Measurements=None
  C2low_ceramic : spsSeriesRLCBranchLib/Series RLC Branch  LConnTagsString=__new0  RConnTagsString=__new0  BranchType=C  Resistance=twist_low_side_rC  Inductance=1e-3  SetiL0=off  InitialCurrent=0  Capacitance=twist_low_side_C_ceramic  Setx0=off  InitialVoltage=source_V  Measurements=None
  C2low_electrolytic : spsSeriesRLCBranchLib/Series RLC Branch  LConnTagsString=__new0  RConnTagsString=__new0  BranchType=RC  Resistance=twist_low_side_rC  Inductance=twist_low_side_lC  SetiL0=off  InitialCurrent=0  Capacitance=twist_low_side_C_electrolytic  Setx0=off  InitialVoltage=source_V  Measurements=None
  Chigh : spsSeriesRLCBranchLib/Series RLC Branch  LConnTagsString=__new0  RConnTagsString=__new0  BranchType=RC  Resistance=twist_high_side_rC  Inductance=1e-3  SetiL0=off  InitialCurrent=0  Capacitance=twist_high_side_C  Setx0=on  InitialVoltage=source_V  Measurements=None
  Controlled Current Source1 : spsControlledCurrentSourceLib/Controlled Current Source  Commented=on  Initialize=on  Source_Type=AC  Amplitude=0  Phase=0  Frequency=0  Measurements=None
  Controlled Current Source2 : spsControlledCurrentSourceLib/Controlled Current Source  Commented=on  Initialize=on  Source_Type=AC  Amplitude=0  Phase=0  Frequency=0  Measurements=None
  Controlled Current Source3 : spsControlledCurrentSourceLib/Controlled Current Source  Commented=on  Initialize=on  Source_Type=AC  Amplitude=0  Phase=0  Frequency=0  Measurements=None
  Current Measurement{,1,5..6} (4 alike) : spsCurrentMeasurementLib/Current Measurement  PhasorSimulation=off  OutputType=Complex  PSBequivalent=0
  From15 : From  Commented=on  GotoTag=QVCC
  From16 : From  Commented=on  GotoTag=i2Loss
  From26 : From  Commented=on  GotoTag=Qjumper
  From28 : From  Commented=on  GotoTag=i1Loss
  From6 : From  Commented=on  GotoTag=feeder_current
  IC : InitialCondition  Value=source_V
  Ideal Switch1 : spsIdealSwitchLib/Ideal Switch  Commented=on  Ron=0.001  Lon=0  IC=0  Rs=1e5  Cs=inf  Measurements=off
  Ideal Switch2 : spsIdealSwitchLib/Ideal Switch  Commented=on  Ron=0.001  Lon=0  IC=0  Rs=1e5  Cs=inf  Measurements=off
  Inductance1 : spsSeriesRLCBranchLib/Series RLC Branch  LConnTagsString=__new0  RConnTagsString=__new0  BranchType=RL  Resistance=twist_low_side_rL  Inductance=twist_low_side_L  SetiL0=off  InitialCurrent=0  Capacitance=1e-6  Setx0=off  InitialVoltage=0  Measurements=None
  Inductance2 : spsSeriesRLCBranchLib/Series RLC Branch  LConnTagsString=__new0  RConnTagsString=__new0  BranchType=RL  Resistance=twist_low_side_rL  Inductance=twist_low_side_L  SetiL0=off  InitialCurrent=0  Capacitance=1e-6  Setx0=off  InitialVoltage=0  Measurements=None
  Meas Feeder : spsSeriesRLCBranchLib/Series RLC Branch  Commented=on  LConnTagsString=__new0  RConnTagsString=__new0  BranchType=R  Resistance=twist_high_side_feeder_R  Inductance=twist_low_side_L  SetiL0=off  InitialCurrent=0  Capacitance=1e-6  Setx0=off  InitialVoltage=0  Measurements=None
  Scope : Scope
  Shottky2 : spsDiodeLib/Diode  Ron=twist_shottky_Ron  Lon=0  Vf=twist_shottky_Vf  IC=0  UseSnubber=0  Rs=twist_shottky_Rs  Cs=twist_shottky_Cs  Measurements=off
  Shottky4 : spsDiodeLib/Diode  Ron=twist_shottky_Ron  Lon=0  Vf=twist_shottky_Vf  IC=0  UseSnubber=0  Rs=twist_shottky_Rs  Cs=twist_shottky_Cs  Measurements=off
  Switch{1..4} (4 alike) : spsMosfetLib/Mosfet  Ron=twist_FET_Ron  Lon=0  Rd=twist_FET_Rd  Vfd=twist_FET_Vf  IC=0  Rs=twist_FET_Rs  Cs=twist_FET_Cs  Measurements=off
  Switch7 : spsMosfetLib/Mosfet  Ron=twist_FET_Clow_Ron  Lon=0  Rd=twist_FET_Clow_Ron  Vfd=0  IC=0  Rs=twist_FET_Rs  Cs=twist_FET_Cs  Measurements=off
  Switch8 : spsMosfetLib/Mosfet  Ron=twist_FET_Clow_Ron  Lon=0  Rd=twist_FET_Clow_Ron  Vfd=0  IC=0  Rs=twist_FET_Rs  Cs=twist_FET_Cs  Measurements=off
  Voltage Measurement : spsVoltageMeasurementLib/Voltage Measurement  PhasorSimulation=off  OutputType=Complex  PSBequivalent=0
  feeder VCC : spsSeriesRLCBranchLib/Series RLC Branch  Commented=on  LConnTagsString=__new0  RConnTagsString=__new0  BranchType=R  Resistance=twist_R_VCC  Inductance=twist_low_side_L  SetiL0=off  InitialCurrent=0  Capacitance=1e-6  Setx0=off  InitialVoltage=0  Measurements=None
  v1Low : spsVoltageMeasurementLib/Voltage Measurement  PhasorSimulation=off  OutputType=Complex  PSBequivalent=0
  v2Low : spsVoltageMeasurementLib/Voltage Measurement  PhasorSimulation=off  OutputType=Complex  PSBequivalent=0
  Load leg2 : PMIOPort  Side=Left
  Load leg1 : PMIOPort  Port=2  Side=Left
  Load GND : PMIOPort  Port=3  Side=Left
  VHigh+ : PMIOPort  Port=4  Side=Right
  VHigh - : PMIOPort  Port=5  Side=Right
  tag scope: i1Meas=global, i2Meas=global, iHMeas=global, i_Chigh=global, v1Meas=global, v2Meas=global, vHMeas=global
  wires:
  From28/1 -> Controlled Current Source3/1
  From6/1 -> Controlled Current Source1/1
  Current Measurement5/1 -> [i2Meas]
  Current Measurement1/1 -> [iHMeas]
  Current Measurement6/1 -> [i1Meas]
  Current Measurement/1 -> [i_Chigh], Scope/1  "i_Chigh"
  [Q1] -> Switch1/1
  [Q3] -> Switch3/1  "Q3"
  IC/1 -> [vHMeas]
  From15/1 -> Ideal Switch2/1
  [Q5] -> Switch7/1
  [Q4] -> Switch4/1  "Q4"
  Voltage Measurement/1 -> IC/1
  v2Low/1 -> [v2Meas]
  [Q6] -> Switch8/1
  From16/1 -> Controlled Current Source2/1
  [Q2] -> Switch2/1
  v1Low/1 -> [v1Meas]
  From26/1 -> Ideal Switch1/1
  connections:
  Inductance2/LConn1 -- Current Measurement5/LConn1
  Current Measurement/RConn1 -- Chigh/LConn1
  VHigh+/RConn1 -- Current Measurement1/LConn1
  Ideal Switch2/LConn1 -- feeder VCC/LConn1
  Meas Feeder/LConn1 -- Ideal Switch1/LConn1
  Load leg1/RConn1 -- ADC Low1/LConn1 -- C1low_electrolytic/LConn1 -- Current Measurement6/RConn1 -- C1low_ceramic/LConn1 -- v1Low/LConn1
  Load leg2/RConn1 -- Current Measurement5/RConn1 -- C2low_ceramic/LConn1 -- C2low_electrolytic/LConn1 -- ADC Low2/LConn1 -- v2Low/LConn1
  Switch3/RConn1 -- Switch4/LConn1 -- Inductance2/RConn1 -- Shottky4/RConn1
  Switch7/LConn1 -- C1low_electrolytic/RConn1
  Ideal Switch1/RConn1 -- Ideal Switch2/RConn1 -- Current Measurement1/RConn1 -- Voltage Measurement/LConn1 -- ADC High/LConn1 -- Current Measurement/LConn1 -- Controlled Current Source1/LConn1 -- Controlled Current Source2/LConn1 -- Switch3/LConn1 -- Switch1/LConn1 -- Controlled Current Source3/LConn1
  Current Measurement6/LConn1 -- Inductance1/LConn1
  Switch8/LConn1 -- C2low_electrolytic/RConn1
  Shottky2/RConn1 -- Inductance1/RConn1 -- Switch1/RConn1 -- Switch2/LConn1
  VHigh -/RConn1 -- Shottky2/LConn1 -- C2low_ceramic/RConn1 -- Switch8/RConn1 -- ADC Low2/RConn1 -- C1low_ceramic/RConn1 -- Switch7/RConn1 -- ADC Low1/RConn1 -- v1Low/LConn2 -- Load GND/RConn1 -- v2Low/LConn2 -- Switch2/RConn1 -- Controlled Current Source3/RConn1 -- Switch4/RConn1 -- Shottky4/LConn1 -- Controlled Current Source2/RConn1 -- Controlled Current Source1/RConn1 -- Chigh/RConn1 -- ADC High/RConn1 -- Meas Feeder/RConn1 -- feeder VCC/RConn1 -- Voltage Measurement/LConn2

== system V1_Grid_Forming_corrected_dq_2022/Subsystem/LEG1 Control  ==
  note: Note 1:
      | All sampling times inferior than Ts = 1e-6 were desactivated or changed to Ts to reduce simulation duration
  note: PWM Timer Model
  note: Note 2:
      | PWM generator original resolution value at 100 ns
  Duty cycle input : Inport
  Activation : Inport  Port=2
  Constant : Constant  Value=0
  Demux : Demux  Outputs=2
  PWM Generator (2-Level) : Subsystem  AncestorBlock=|  DialogController=POWERSYS.PowerSysDialog  LoadFcn=sps_rtmsupport('LoadFcn', gcbh);  StartFcn=sps_rtmsupport('StartFcn', gcbh);  StopFcn=sps_rtmsupport('StopFcn', gcbh);  BlockChoice=InternalUref  mask(PWM Generator (2-Level)){ModulatorType=Single-phase half-bridge (2 pulses), ModulatorMode=Unsynchronized, Fc=twist_freq_switching, Pc=0, nF=27, MinMax=[0 1], SamplingTechnique=Symmetrical regular (single edge), ModulatingSignals=off, m=0.8, Freq=60, Phase=0, Ts=Ts, ShowCarrierOutport=off}
      | spsPWMGenerator2LevelLib/PWM Generator
      | (2-Level)
      mask prompts: ModulatorType "Generator type:"; ModulatorMode "Mode of operation:"; Fc "Frequency (Hz):"; Pc "Initial phase (degrees):"; nF "Switching ratio (carrier frequency / output frequency):"; MinMax "Minimum and maximum values: [ Min  Max ]"; SamplingTechnique "Sampling technique:"; ModulatingSignals "Internal generation of reference signal"; m "Modulation index:"; Freq "Frequency (Hz):"; Phase "Phase (degrees):"; Ts "Sample time (s):"; ShowCarrierOutport "Show measurement port"
      mask help:
      | Generate pulses for PWM-controlled 2-Level converter, using carrier-based two-level PWM method. The block can control switching devices of single-phase half-bridge, single-phase full-bridge (unipolar or bipolar modulation) or three-phase bridge.
      |
      | When the Synchronized mode of operation is selected, a second input is added to the block, and the internal generation of modulating signal is disabled. Use input 2 (wt) to synchronize the carrier.
      mask init:
      | sps = powericon('PWMGenerator2LevelInit',gcb,ModulatorType,SamplingTechnique,ModulatorMode,nF,Fc,MinMax,Pc,ShowCarrierOutport,ModulatingSignals,m,Freq,Phase,Ts);
      settings: CopyFcn=sps_rtmsupport('CopyFcn', gcbh);  DeleteFcn=sps_rtmsupport('DeleteFcn', gcbh);  UndoDeleteFcn=sps_rtmsupport('UndoDeleteFcn', gcbh);  ModelCloseFcn=sps_rtmsupport('ModelCloseFcn', gcbh);  PreSaveFcn=sps_rtmsupport('PreSaveFcn', gcbh);  PostSaveFcn=sps_rtmsupport('PostSaveFcn', gcbh);  NameChangeFcn=sps_rtmsupport('NameChangeFcn', gcbh);  PreCopyFcn=sps_rtmsupport('PreCopyFcn', gcbh);  OpenFcn="sps_rtmsupport('OpenFcn', gcbh, [1   2   7   8  13]);"  CloseFcn=sps_rtmsupport('CloseFcn', gcbh);  PreDeleteFcn=sps_rtmsupport('PreDeleteFcn', gcbh);
      settings: LibrarySourceBlock=|
      | spsPWMGenerator2LevelLib/PWM Generator
      | (2-Level)
      mask Help: helpview(psbhelp);
      mask TypeOptions ModulatorType: Single-phase half-bridge (2 pulses) | Single-phase full-bridge (4 pulses) | Single-phase full-bridge - Bipolar modulation (4 pulses) | Three-phase bridge (6 pulses)
      mask TypeOptions ModulatorMode: Synchronized | Unsynchronized
      mask Callback ModulatorMode: powericon('PWMGenerator2LevelCback',gcb);
      mask TypeOptions SamplingTechnique: Natural | Asymmetrical regular (double edge) | Symmetrical regular (single edge)
      mask Callback ModulatingSignals: powericon('PWMGenerator2LevelCback',gcb);
      mask DialogControl Container3 Prompt: Carrier
      mask DialogControl ModulatingSignalParameters Prompt: Reference signal
  Switch : Switch  Criteria=u2 > Threshold  SaturateOnIntegerOverflow=off  InputSameDT=off
  Switch1 : Switch  Criteria=u2 > Threshold  SaturateOnIntegerOverflow=off  InputSameDT=off
  High-Side Q : Outport
  Low-Side Q : Outport  Port=2
  Carry Leg : Outport  Port=3
  wires:
  Switch1/1 -> Low-Side Q/1
  PWM Generator (2-Level)/1(P) -> Demux/1  "PWM_out"
  Demux/1 -> Switch/1  "high side"
  PWM Generator (2-Level)/2(Carry) -> Carry Leg/1  "carrier"
  Activation/1 -> Switch/2, Switch1/2
  Switch/1 -> High-Side Q/1
  Demux/2 -> Switch1/1  "low side"
  Duty cycle input/1 -> PWM Generator (2-Level)/1(Uref)
  Constant/1 -> Switch1/3, Switch/3

== system V1_Grid_Forming_corrected_dq_2022/Subsystem/LEG2 Control ==
  note: Note 2:
      | PWM generator original resolution value at 100 ns
  note: PWM Timer Model
  note: Note 1:
      | All sampling times inferior than Ts = 1e-6 were desactivated or changed to Ts to reduce simulation duration
  Duty cycle input : Inport
  Activation : Inport  Port=2
  Constant : Constant  Value=0
  Demux : Demux  Outputs=2
  PWM Generator (2-Level) : Subsystem  AncestorBlock=|  DialogController=POWERSYS.PowerSysDialog  LoadFcn=sps_rtmsupport('LoadFcn', gcbh);  StartFcn=sps_rtmsupport('StartFcn', gcbh);  StopFcn=sps_rtmsupport('StopFcn', gcbh);  BlockChoice=InternalUref  mask(PWM Generator (2-Level)){ModulatorType=Single-phase half-bridge (2 pulses), ModulatorMode=Unsynchronized, Fc=twist_freq_switching, Pc=0, nF=27, MinMax=[0 1], SamplingTechnique=Symmetrical regular (single edge), ModulatingSignals=off, m=0.8, Freq=60, Phase=0, Ts=Ts, ShowCarrierOutport=off}
      | spsPWMGenerator2LevelLib/PWM Generator
      | (2-Level)
      mask prompts: ModulatorType "Generator type:"; ModulatorMode "Mode of operation:"; Fc "Frequency (Hz):"; Pc "Initial phase (degrees):"; nF "Switching ratio (carrier frequency / output frequency):"; MinMax "Minimum and maximum values: [ Min  Max ]"; SamplingTechnique "Sampling technique:"; ModulatingSignals "Internal generation of reference signal"; m "Modulation index:"; Freq "Frequency (Hz):"; Phase "Phase (degrees):"; Ts "Sample time (s):"; ShowCarrierOutport "Show measurement port"
      mask help:
      | Generate pulses for PWM-controlled 2-Level converter, using carrier-based two-level PWM method. The block can control switching devices of single-phase half-bridge, single-phase full-bridge (unipolar or bipolar modulation) or three-phase bridge.
      |
      | When the Synchronized mode of operation is selected, a second input is added to the block, and the internal generation of modulating signal is disabled. Use input 2 (wt) to synchronize the carrier.
      mask init:
      | sps = powericon('PWMGenerator2LevelInit',gcb,ModulatorType,SamplingTechnique,ModulatorMode,nF,Fc,MinMax,Pc,ShowCarrierOutport,ModulatingSignals,m,Freq,Phase,Ts);
      settings: CopyFcn=sps_rtmsupport('CopyFcn', gcbh);  DeleteFcn=sps_rtmsupport('DeleteFcn', gcbh);  UndoDeleteFcn=sps_rtmsupport('UndoDeleteFcn', gcbh);  ModelCloseFcn=sps_rtmsupport('ModelCloseFcn', gcbh);  PreSaveFcn=sps_rtmsupport('PreSaveFcn', gcbh);  PostSaveFcn=sps_rtmsupport('PostSaveFcn', gcbh);  NameChangeFcn=sps_rtmsupport('NameChangeFcn', gcbh);  PreCopyFcn=sps_rtmsupport('PreCopyFcn', gcbh);  OpenFcn="sps_rtmsupport('OpenFcn', gcbh, [1   2   7   8  13]);"  CloseFcn=sps_rtmsupport('CloseFcn', gcbh);  PreDeleteFcn=sps_rtmsupport('PreDeleteFcn', gcbh);
      settings: LibrarySourceBlock=|
      | spsPWMGenerator2LevelLib/PWM Generator
      | (2-Level)
      mask Help: helpview(psbhelp);
      mask TypeOptions ModulatorType: Single-phase half-bridge (2 pulses) | Single-phase full-bridge (4 pulses) | Single-phase full-bridge - Bipolar modulation (4 pulses) | Three-phase bridge (6 pulses)
      mask TypeOptions ModulatorMode: Synchronized | Unsynchronized
      mask Callback ModulatorMode: powericon('PWMGenerator2LevelCback',gcb);
      mask TypeOptions SamplingTechnique: Natural | Asymmetrical regular (double edge) | Symmetrical regular (single edge)
      mask Callback ModulatingSignals: powericon('PWMGenerator2LevelCback',gcb);
      mask DialogControl Container3 Prompt: Carrier
      mask DialogControl ModulatingSignalParameters Prompt: Reference signal
  Switch : Switch  Criteria=u2 > Threshold  SaturateOnIntegerOverflow=off  InputSameDT=off
  Switch1 : Switch  Criteria=u2 > Threshold  SaturateOnIntegerOverflow=off  InputSameDT=off
  High-Side Q : Outport
  Low-Side Q : Outport  Port=2
  Carry Leg : Outport  Port=3
  wires:
  Constant/1 -> Switch/3, Switch1/3
  Duty cycle input/1 -> PWM Generator (2-Level)/1(Uref)
  Demux/2 -> Switch1/1  "low side"
  Switch/1 -> High-Side Q/1
  Activation/1 -> Switch1/2, Switch/2
  PWM Generator (2-Level)/2(Carry) -> Carry Leg/1  "carrier"
  Demux/1 -> Switch/1  "high side"
  PWM Generator (2-Level)/1(P) -> Demux/1  "PWM_out"
  Switch1/1 -> Low-Side Q/1

== system V1_Grid_Forming_corrected_dq_2022/Subsystem1/i1Low acquisition ==
  In1 : Inport
  In2 : Inport  Port=2
  If : If  IfExpression=u1 > 0.99  ShowElse=off
  If Action Subsystem : Subsystem  TreatAsAtomicUnit=on
  Scope : Scope  NumInputPorts=3
  i1Meas : Outport
  wires:
  If Action Subsystem/1(Out1) -> Scope/1, i1Meas/1  "Data_Carry"
  In1/1 -> Scope/2, If Action Subsystem/1(In1)  "Data"
  If/1 -> If Action Subsystem/Action
  In2/1 -> If/1, Scope/3  "Carry"

== system V1_Grid_Forming_corrected_dq_2022/Subsystem1/i2Low acquisition ==
  In1 : Inport
  In2 : Inport  Port=2
  If : If  IfExpression=u1 > 0.99  ShowElse=off
  If Action Subsystem : Subsystem  TreatAsAtomicUnit=on
  Scope : Scope  NumInputPorts=3
  i2Meas : Outport
  wires:
  If Action Subsystem/1(Out1) -> Scope/1, i2Meas/1  "Data_Carry"
  In1/1 -> Scope/2, If Action Subsystem/1(In1)  "Data"
  If/1 -> If Action Subsystem/Action
  In2/1 -> If/1, Scope/3  "Carry"

== system V1_Grid_Forming_corrected_dq_2022/Subsystem1/iHigh acquisition ==
  In1 : Inport
  In2 : Inport  Port=2
  If : If  IfExpression=u1 > 0.99  ShowElse=off
  If Action Subsystem : Subsystem  TreatAsAtomicUnit=on
  Scope : Scope  NumInputPorts=3
  iHMeas : Outport
  wires:
  If Action Subsystem/1(Out1) -> Scope/1, iHMeas/1  "Data_Carry"
  In1/1 -> Scope/2, If Action Subsystem/1(In1)  "Data"
  If/1 -> If Action Subsystem/Action
  In2/1 -> If/1, Scope/3  "Carry"

== system V1_Grid_Forming_corrected_dq_2022/Subsystem1/v1Low acquisition ==
  In1 : Inport
  In2 : Inport  Port=2
  If : If  IfExpression=u1 > 0.99  ShowElse=off
  If Action Subsystem : Subsystem  TreatAsAtomicUnit=on
  Scope : Scope  NumInputPorts=3
  v1Meas : Outport
  wires:
  If Action Subsystem/1(Out1) -> Scope/1, v1Meas/1  "Data_Carry"
  In1/1 -> Scope/2, If Action Subsystem/1(In1)  "Data"
  If/1 -> If Action Subsystem/Action
  In2/1 -> If/1, Scope/3  "Carry"

== system V1_Grid_Forming_corrected_dq_2022/Subsystem1/v2Low acquisition ==
  In1 : Inport
  In2 : Inport  Port=2
  If : If  IfExpression=u1 > 0.99  ShowElse=off
  If Action Subsystem : Subsystem  TreatAsAtomicUnit=on
  Scope : Scope  NumInputPorts=3
  v2Meas : Outport
  wires:
  If Action Subsystem/1(Out1) -> Scope/1, v2Meas/1  "Data_Carry"
  In1/1 -> Scope/2, If Action Subsystem/1(In1)  "Data"
  If/1 -> If Action Subsystem/Action
  In2/1 -> If/1, Scope/3  "Carry"

== system V1_Grid_Forming_corrected_dq_2022/Subsystem1/vHigh acquisition ==
  In1 : Inport
  In2 : Inport  Port=2
  If : If  IfExpression=u1 > 0.99  ShowElse=off
  If Action Subsystem : Subsystem  TreatAsAtomicUnit=on
  Scope : Scope  NumInputPorts=3
  vHMeas : Outport
  wires:
  If Action Subsystem/1(Out1) -> Scope/1, vHMeas/1  "Data_Carry"
  In1/1 -> Scope/2, If Action Subsystem/1(In1)  "Data"
  If/1 -> If Action Subsystem/Action
  In2/1 -> If/1, Scope/3  "Carry"
